simulink model "sampleModel7126_pp_1_1"  (R2018a)
settings: Solver=VariableStepAuto  StartTime=0.0  StopTime=10.0  RelTol=1e-3
undefined symbols (not defined in the file): DiscIntNeverNeededParam
libraries: simulink x367
(part 5 of 12)

== system sampleModel7126_pp_1_1/cfblk284 ==
  cfblk1 : Inport
  cfblk8 : Inport  Port=2
  Action Port : ActionPort  ActionType=else
  cfblk10 : Subsystem  TreatAsAtomicUnit=on
  cfblk11 : Subsystem  TreatAsAtomicUnit=on
  cfblk12 : Subsystem  TreatAsAtomicUnit=on
  cfblk{5,13..14,16} (4 alike) : Delay
  cfblk15 : Subsystem  TreatAsAtomicUnit=on
  cfblk3 : Subsystem  TreatAsAtomicUnit=on
  cfblk4 : simulink/Continuous/PID Controller (2DOF)  Controller=PID  TimeDomain=Discrete-time  SampleTime=-1  IntegratorMethod=Forward Euler  FilterMethod=Forward Euler  Form=Parallel  UseFilter=on  ControllerParametersSource=internal  P=1  I=1  D=0  N=100  b=1  c=1  InitialConditionSource=internal  InitialConditionForIntegrator=0  InitialConditionForFilter=0  ExternalReset=none  LimitOutput=off  UpperSaturationLimit=inf  LowerSaturationLimit=-inf  LinearizeAsGain=off  AntiWindupMode=none  Kb=1  TrackingMode=off  Kt=1  PParamMin=[]  PParamMax=[]  IParamMin=[]  IParamMax=[]  DParamMin=[]  DParamMax=[]  NParamMin=[]  NParamMax=[]  bParamMin=[]  bParamMax=[]  cParamMin=[]  cParamMax=[]  KbParamMin=[]  KbParamMax=[]  KtParamMin=[]  KtParamMax=[]  POutMin=[]  POutMax=[]  IOutMin=[]  IOutMax=[]  DOutMin=[]  DOutMax=[]  NOutMin=[]  NOutMax=[]  bOutMin=[]  bOutMax=[]  cOutMin=[]  cOutMax=[]  KbOutMin=[]  KbOutMax=[]  KtOutMin=[]  KtOutMax=[]  IntegratorOutMin=[]  IntegratorOutMax=[]  FilterOutMin=[]  FilterOutMax=[]  SumOutMin=[]  SumOutMax=[]  Sum1OutMin=[]  Sum1OutMax=[]  Sum2OutMin=[]  Sum2OutMax=[]  Sum3OutMin=[]  Sum3OutMax=[]  SumI1OutMin=[]  SumI1OutMax=[]  SumI2OutMin=[]  SumI2OutMax=[]  SumI3OutMin=[]  SumI3OutMax=[]  SumDOutMin=[]  SumDOutMax=[]  SaturationOutMin=[]  SaturationOutMax=[]  IntegratorContinuousStateAttributes=''  IntegratorStateMustResolveToSignalObject=off  IntegratorRTWStateStorageClass=Auto  FilterContinuousStateAttributes=''  FilterStateMustResolveToSignalObject=off  FilterRTWStateStorageClass=Auto  DifferentiatorICPrevScaledInput=0  DifferentiatorOutMin=[]  DifferentiatorOutMax=[]  FilterDiffOutCoefMin=[]  FilterDiffOutCoefMax=[]  SumDenOutMin=[]  SumDenOutMax=[]  SumNumOutMin=[]  SumNumOutMax=[]  ReciprocalOutMin=[]  ReciprocalOutMax=[]  DivideOutMin=[]  DivideOutMax=[]  TunerSelectOption=Transfer Function Based (PID Tuner App)
  cfblk6 : Delay  DelayLengthSource=Input port
      settings: InputPortMap=u0,p1
  cfblk7 : If  SampleTime=1
  cyemi_{1015..1018,1026..1028,1043..1054} (19 alike) : DataTypeConversion  OutDataTypeStr=double
  emi_1219 : Subsystem  TreatAsAtomicUnit=on
  emi_1221 : If  IfExpression=0 <= u1
  emi_1222 : DataTypeConversion  OutDataTypeStr=double
  emi_1655 : Subsystem  TreatAsAtomicUnit=on
  emi_1657 : If  IfExpression=0 <= u1  SampleTime=[1 0]
  emi_1658 : DataTypeConversion  OutDataTypeStr=double
  emi_2001 : Subsystem  TreatAsAtomicUnit=on
  emi_2003 : If  IfExpression=0 <= u1  SampleTime=[1 0]
  emi_2004 : DataTypeConversion  OutDataTypeStr=double
  cfblk2 : Outport
  cfblk9 : Outport  Port=2
  wires:
  cfblk8/1 -> cyemi_1016/1, cyemi_1048/1
  cfblk5/1 -> cfblk2/1, cyemi_1044/1, emi_1222/1
  cfblk4/1 -> cyemi_1043/1, cyemi_1046/1, cyemi_1047/1
  cfblk10/2(cfblk13) -> cfblk9/1
  cfblk7/1 -> cfblk10/Action
  cfblk7/2 -> cfblk11/Action
  cyemi_1015/1 -> cfblk10/1(cfblk1)
  cfblk14/1 -> cyemi_1015/1
  cyemi_1016/1 -> cfblk10/2(cfblk10)
  cyemi_1017/1 -> cfblk10/3(cfblk11)
  cfblk16/1 -> cyemi_1017/1
  cyemi_1018/1 -> cfblk10/4(cfblk12)
  cfblk13/1 -> cyemi_1018/1
  cyemi_1026/1 -> cfblk11/1(cfblk1)
  cyemi_1027/1 -> cfblk11/2(cfblk13)
  cfblk10/4(cfblk15) -> cyemi_1027/1
  cyemi_1028/1 -> cfblk11/3(cfblk14)
  cyemi_1044/1 -> cfblk13/1
  cyemi_1045/1 -> cfblk14/1
  cfblk11/2(cfblk15) -> cyemi_1045/1
  cyemi_1047/1 -> cfblk16/1
  cyemi_1049/1 -> cfblk4/1
  cfblk10/1(cfblk2) -> cyemi_1049/1
  cyemi_1050/1 -> cfblk4/2
  cfblk10/3(cfblk14) -> cyemi_1050/1
  cyemi_1051/1 -> cfblk5/1
  cfblk6/1 -> cyemi_1051/1, emi_1658/1, emi_2004/1
  cyemi_1052/1 -> cfblk6/1
  cyemi_1053/1 -> cfblk6/2
  cfblk11/1(cfblk2) -> cyemi_1053/1
  cyemi_1054/1 -> cfblk7/1
  cfblk1/1 -> cyemi_1054/1
  cyemi_1043/1 -> cfblk12/1(emi_1217)
  cfblk12/1(emi_1218) -> cyemi_1026/1
  emi_1221/1 -> cfblk12/Action
  emi_1221/2 -> emi_1219/Action
  emi_1222/1 -> emi_1221/1
  cyemi_1048/1 -> cfblk3/1(emi_1653)
  cfblk3/1(emi_1654) -> cyemi_1052/1
  emi_1657/1 -> cfblk3/Action
  emi_1657/2 -> emi_1655/Action
  emi_1658/1 -> emi_1657/1
  cyemi_1046/1 -> cfblk15/1(emi_1999)
  cfblk15/1(emi_2000) -> cyemi_1028/1
  emi_2003/1 -> cfblk15/Action
  emi_2003/2 -> emi_2001/Action
  emi_2004/1 -> emi_2003/1

== system sampleModel7126_pp_1_1/cfblk285 ==
  cfblk1 : Inport
  cfblk8 : Inport  Port=2
  cfblk9 : Inport  Port=3
  Action Port : ActionPort  ActionType=then
  cfblk3 : DiscreteZeroPole  Poles=[0 0.5]  Gain=1  SampleTime=-1
  cfblk4 : simulink/Discrete/Tapped Delay  vinit=0.0  samptime=-1  NumDelays=1  DelayOrder=Oldest  includeCurrent=off
  cfblk5 : simulink/Discrete/Transfer Fcn Lead or Lag  PoleZ=0.95  ZeroZ=0.75  ICPrevOutput=0.0  ICPrevInput=0.0  DoSatur=off
      settings: SourceProductName=Simulink  SourceProductBaseCode=SL
  cfblk6 : Subsystem  TreatAsAtomicUnit=on
  cfblk7 : DiscreteTransferFcn
  cyemi_{1058..1062} (5 alike) : DataTypeConversion  OutDataTypeStr=double
  emi_762 : Subsystem  TreatAsAtomicUnit=on
  emi_764 : If  IfExpression=Inf <= u1  SampleTime=[1 0]
  emi_765 : DataTypeConversion  OutDataTypeStr=double
  cfblk2 : Outport
  wires:
  cfblk3/1 -> cfblk2/1, emi_765/1
  cyemi_1058/1 -> cfblk3/1
  cyemi_1059/1 -> cfblk4/1
  cfblk7/1 -> cyemi_1059/1
  cyemi_1060/1 -> cfblk5/1
  cfblk1/1 -> cyemi_1060/1
  cfblk9/1 -> cyemi_1061/1
  cyemi_1062/1 -> cfblk7/1
  cfblk5/1 -> cyemi_1062/1
  cyemi_1061/1 -> cfblk6/1(emi_760)
  cfblk6/1(emi_761) -> cyemi_1058/1
  emi_764/1 -> cfblk6/Action
  emi_764/2 -> emi_762/Action
  emi_765/1 -> emi_764/1

== system sampleModel7126_pp_1_1/cfblk286 ==
  cfblk1 : Inport
  cfblk7 : Inport  Port=2
  cfblk8 : Inport  Port=3
  Action Port : ActionPort  ActionType=else
  cfblk3 : simulink/Discrete/Difference  ICPrevInput=0.0  OutMin=[]  OutMax=[]  OutDataTypeStr=double  OutputDataTypeScalingMode=double  OutDataType=fixdt(1, 16)  OutScaling=2^-10  DoSatur=off
  cfblk4 : UnitDelay  SampleTime=-1
  cfblk5 : Subsystem  TreatAsAtomicUnit=on
  cfblk6 : DiscreteStateSpace  SampleTime=-1
  cyemi_1066 : DataTypeConversion  OutDataTypeStr=double
  cyemi_1067 : DataTypeConversion  OutDataTypeStr=uint8
  cyemi_1068 : DataTypeConversion  OutDataTypeStr=double
  cyemi_1069 : DataTypeConversion  OutDataTypeStr=double
  emi_734 : Subsystem  TreatAsAtomicUnit=on
  emi_736 : If  IfExpression=0 <= u1  SampleTime=[1 0]
  emi_737 : DataTypeConversion  OutDataTypeStr=uint8
  cfblk2 : Outport
  wires:
  cfblk4/1 -> cfblk2/1, emi_737/1
  cyemi_1066/1 -> cfblk3/1
  cyemi_1067/1 -> cfblk4/1
  cfblk1/1 -> cyemi_1067/1
  cfblk8/1 -> cyemi_1068/1
  cyemi_1069/1 -> cfblk6/1
  cfblk7/1 -> cyemi_1069/1
  cyemi_1068/1 -> cfblk5/1(emi_732)
  cfblk5/1(emi_733) -> cyemi_1066/1
  emi_736/1 -> cfblk5/Action
  emi_736/2 -> emi_734/Action
  emi_737/1 -> emi_736/1

== system sampleModel7126_pp_1_1/cfblk287 ==
  cfblk1 : Inport
  cfblk8 : Inport  Port=2
  cfblk9 : Inport  Port=3
  Action Port : ActionPort  ActionType=then
  cfblk10 : Delay
  cfblk3 : simulink/Continuous/PID Controller (2DOF)  Controller=PID  TimeDomain=Discrete-time  SampleTime=-1  IntegratorMethod=Forward Euler  FilterMethod=Forward Euler  Form=Parallel  UseFilter=on  ControllerParametersSource=internal  P=1  I=1  D=0  N=100  b=1  c=1  InitialConditionSource=internal  InitialConditionForIntegrator=0  InitialConditionForFilter=0  ExternalReset=none  LimitOutput=off  UpperSaturationLimit=inf  LowerSaturationLimit=-inf  LinearizeAsGain=off  AntiWindupMode=none  Kb=1  TrackingMode=off  Kt=1  PParamMin=[]  PParamMax=[]  IParamMin=[]  IParamMax=[]  DParamMin=[]  DParamMax=[]  NParamMin=[]  NParamMax=[]  bParamMin=[]  bParamMax=[]  cParamMin=[]  cParamMax=[]  KbParamMin=[]  KbParamMax=[]  KtParamMin=[]  KtParamMax=[]  POutMin=[]  POutMax=[]  IOutMin=[]  IOutMax=[]  DOutMin=[]  DOutMax=[]  NOutMin=[]  NOutMax=[]  bOutMin=[]  bOutMax=[]  cOutMin=[]  cOutMax=[]  KbOutMin=[]  KbOutMax=[]  KtOutMin=[]  KtOutMax=[]  IntegratorOutMin=[]  IntegratorOutMax=[]  FilterOutMin=[]  FilterOutMax=[]  SumOutMin=[]  SumOutMax=[]  Sum1OutMin=[]  Sum1OutMax=[]  Sum2OutMin=[]  Sum2OutMax=[]  Sum3OutMin=[]  Sum3OutMax=[]  SumI1OutMin=[]  SumI1OutMax=[]  SumI2OutMin=[]  SumI2OutMax=[]  SumI3OutMin=[]  SumI3OutMax=[]  SumDOutMin=[]  SumDOutMax=[]  SaturationOutMin=[]  SaturationOutMax=[]  IntegratorContinuousStateAttributes=''  IntegratorStateMustResolveToSignalObject=off  IntegratorRTWStateStorageClass=Auto  FilterContinuousStateAttributes=''  FilterStateMustResolveToSignalObject=off  FilterRTWStateStorageClass=Auto  DifferentiatorICPrevScaledInput=0  DifferentiatorOutMin=[]  DifferentiatorOutMax=[]  FilterDiffOutCoefMin=[]  FilterDiffOutCoefMax=[]  SumDenOutMin=[]  SumDenOutMax=[]  SumNumOutMin=[]  SumNumOutMax=[]  ReciprocalOutMin=[]  ReciprocalOutMax=[]  DivideOutMin=[]  DivideOutMax=[]  TunerSelectOption=Transfer Function Based (PID Tuner App)
  cfblk4 : Subsystem  TreatAsAtomicUnit=on
  cfblk5 : DiscreteIntegrator  SampleTime=-1  OutDataTypeStr=double  ICPrevOutput=DiscIntNeverNeededParam  ICPrevScaledInput=DiscIntNeverNeededParam
  cfblk6 : Subsystem  TreatAsAtomicUnit=on
  cfblk7 : Subsystem  TreatAsAtomicUnit=on
  cyemi_{1073..1080} (8 alike) : DataTypeConversion  OutDataTypeStr=double
  emi_1677 : Subsystem  TreatAsAtomicUnit=on
  emi_1679 : If  IfExpression=Inf <= u1  SampleTime=[1 0]
  emi_1680 : DataTypeConversion  OutDataTypeStr=double
  emi_720 : Subsystem  TreatAsAtomicUnit=on
  emi_722 : If  IfExpression=Inf <= u1  SampleTime=[1 0]
  emi_723 : DataTypeConversion  OutDataTypeStr=double
  emi_755 : Subsystem  TreatAsAtomicUnit=on
  emi_757 : If  IfExpression=Inf <= u1  SampleTime=[1 0]
  emi_758 : DataTypeConversion  OutDataTypeStr=double
  cfblk2 : Outport
  wires:
  cfblk5/1 -> cfblk2/1, emi_1680/1
  cyemi_1073/1 -> cfblk10/1
  cyemi_1074/1 -> cfblk3/1
  cfblk10/1 -> cyemi_1074/1
  cyemi_1075/1 -> cfblk3/2
  cfblk9/1 -> cyemi_1075/1
  cfblk3/1 -> cyemi_1076/1
  cyemi_1077/1 -> cfblk5/1
  cfblk1/1 -> cyemi_1078/1
  cfblk8/1 -> cyemi_1080/1
  cyemi_1076/1 -> cfblk4/1(emi_718)
  cfblk4/1(emi_719) -> cyemi_1073/1
  emi_722/1 -> cfblk4/Action
  emi_722/2 -> emi_720/Action
  emi_723/1 -> emi_722/1
  cyemi_1078/1 -> cfblk6/1(emi_753)
  cfblk6/1(emi_754) -> cyemi_1079/1
  emi_757/1 -> cfblk6/Action
  emi_757/2 -> emi_755/Action
  emi_758/1 -> emi_757/1
  cyemi_1079/1 -> cfblk7/1(emi_1674)
  cyemi_1080/1 -> cfblk7/2(emi_1675)
  cfblk7/1(emi_1676) -> emi_758/1, emi_723/1, cyemi_1077/1
  emi_1679/1 -> cfblk7/Action
  emi_1679/2 -> emi_1677/Action
  emi_1680/1 -> emi_1679/1

== system sampleModel7126_pp_1_1/cfblk288 ==
  cfblk1 : Inport
  cfblk13 : Inport  Port=2
  Action Port : ActionPort  ActionType=else
  cfblk10 : simulink/Discrete/Tapped Delay  vinit=0.0  samptime=-1  NumDelays=1  DelayOrder=Oldest  includeCurrent=off
  cfblk11 : Subsystem  TreatAsAtomicUnit=on
  cfblk12 : DiscreteStateSpace  SampleTime=-1
  cfblk3 : Subsystem  TreatAsAtomicUnit=on
  cfblk4 : UnitDelay  SampleTime=-1
  cfblk5 : DiscreteFir
  cfblk6 : Delay  ShowEnablePort=on
      settings: InputPortMap=u0,e6
  cfblk7 : simulink/Discrete/Transfer Fcn First Order  PoleZ=0.95  ICPrevOutput=0.0  DoSatur=off
      settings: SourceProductName=Simulink
  cfblk8 : simulink/Continuous/PID Controller  Controller=PID  TimeDomain=Discrete-time  SampleTime=-1  IntegratorMethod=Forward Euler  FilterMethod=Forward Euler  Form=Parallel  UseFilter=on  ControllerParametersSource=internal  P=1  I=1  D=0  N=100  InitialConditionSource=internal  InitialConditionForIntegrator=0  InitialConditionForFilter=0  ExternalReset=none  LimitOutput=off  UpperSaturationLimit=inf  LowerSaturationLimit=-inf  LinearizeAsGain=off  AntiWindupMode=none  Kb=1  TrackingMode=off  Kt=1  PParamMin=[]  PParamMax=[]  IParamMin=[]  IParamMax=[]  DParamMin=[]  DParamMax=[]  NParamMin=[]  NParamMax=[]  KbParamMin=[]  KbParamMax=[]  KtParamMin=[]  KtParamMax=[]  POutMin=[]  POutMax=[]  IOutMin=[]  IOutMax=[]  DOutMin=[]  DOutMax=[]  NOutMin=[]  NOutMax=[]  KbOutMin=[]  KbOutMax=[]  KtOutMin=[]  KtOutMax=[]  IntegratorOutMin=[]  IntegratorOutMax=[]  FilterOutMin=[]  FilterOutMax=[]  SumOutMin=[]  SumOutMax=[]  SumI1OutMin=[]  SumI1OutMax=[]  SumI2OutMin=[]  SumI2OutMax=[]  SumI3OutMin=[]  SumI3OutMax=[]  SumDOutMin=[]  SumDOutMax=[]  SaturationOutMin=[]  SaturationOutMax=[]  IntegratorContinuousStateAttributes=''  IntegratorStateMustResolveToSignalObject=off  IntegratorRTWStateStorageClass=Auto  FilterContinuousStateAttributes=''  FilterStateMustResolveToSignalObject=off  FilterRTWStateStorageClass=Auto  DifferentiatorICPrevScaledInput=0  DifferentiatorOutMin=[]  DifferentiatorOutMax=[]  FilterDiffOutCoefMin=[]  FilterDiffOutCoefMax=[]  SumDenOutMin=[]  SumDenOutMax=[]  SumNumOutMin=[]  SumNumOutMax=[]  ReciprocalOutMin=[]  ReciprocalOutMax=[]  DivideOutMin=[]  DivideOutMax=[]  TunerSelectOption=Transfer Function Based (PID Tuner App)
  cfblk9 : DiscreteTransferFcn
  cyemi_{1083..1093} (11 alike) : DataTypeConversion  OutDataTypeStr=double
  emi_1350 : Subsystem  TreatAsAtomicUnit=on
  emi_1352 : If  IfExpression=0 <= u1  SampleTime=[1 0]
  emi_1353 : DataTypeConversion  OutDataTypeStr=double
  emi_346 : Subsystem  TreatAsAtomicUnit=on
  emi_348 : If  IfExpression=0 <= u1  SampleTime=[1 0]
  emi_349 : DataTypeConversion  OutDataTypeStr=double
  cfblk2 : Outport
  wires:
  cfblk12/1 -> cfblk2/1
  cyemi_1083/1 -> cfblk10/1
  cfblk8/1 -> cyemi_1083/1
  cfblk4/1 -> cyemi_1084/1
  cyemi_1085/1 -> cfblk12/1
  cfblk6/1 -> cyemi_1086/1, emi_349/1
  cyemi_1087/1 -> cfblk4/1
  cfblk7/1 -> cyemi_1087/1
  cyemi_1088/1 -> cfblk5/1
  cyemi_1089/1 -> cfblk6/1
  cfblk1/1 -> cyemi_1089/1
  cyemi_1090/1 -> cfblk6/2
  cfblk13/1 -> cyemi_1090/1
  cyemi_1091/1 -> cfblk7/1
  cfblk9/1 -> cyemi_1091/1
  cyemi_1092/1 -> cfblk8/1
  cfblk5/1 -> cyemi_1092/1
  cyemi_1093/1 -> cfblk9/1
  cfblk10/1 -> cyemi_1093/1, emi_1353/1
  cyemi_1084/1 -> cfblk11/1(emi_344)
  cfblk11/1(emi_345) -> cyemi_1085/1
  emi_348/1 -> cfblk11/Action
  emi_348/2 -> emi_346/Action
  emi_349/1 -> emi_348/1
  cyemi_1086/1 -> cfblk3/1(emi_1348)
  cfblk3/1(emi_1349) -> cyemi_1088/1
  emi_1352/1 -> cfblk3/Action
  emi_1352/2 -> emi_1350/Action
  emi_1353/1 -> emi_1352/1

== system sampleModel7126_pp_1_1/cfblk289 ==
  cfblk1 : Inport
  Action Port : ActionPort  ActionType=then
  cfblk10 : Subsystem  TreatAsAtomicUnit=on
  cfblk11 : Subsystem  TreatAsAtomicUnit=on
  cfblk12 : Delay
  cfblk3 : simulink/Discrete/Transfer Fcn First Order  PoleZ=0.95  ICPrevOutput=0.0  DoSatur=off
      settings: SourceProductName=Simulink
  cfblk4 : DiscreteStateSpace  SampleTime=-1
  cfblk5 : simulink/Discrete/Transfer Fcn Real Zero  ZeroZ=0.75  ICPrevInput=0.0  DoSatur=off
      settings: SourceProductName=Simulink  SourceProductBaseCode=SL
  cfblk6 : DiscreteZeroPole  Poles=[0 0.5]  Gain=1  SampleTime=-1
  cfblk7 : If  SampleTime=1
  cfblk9 : Subsystem  TreatAsAtomicUnit=on
  cyemi_{1095..1096,1108..1116} (11 alike) : DataTypeConversion  OutDataTypeStr=double
  emi_1126 : Subsystem  TreatAsAtomicUnit=on
  emi_1128 : If  IfExpression=Inf <= u1
  emi_1129 : DataTypeConversion  OutDataTypeStr=double
  cfblk2 : Outport
  cfblk8 : Outport  Port=2
  wires:
  cfblk4/1 -> cyemi_1114/1, cyemi_1115/1, cyemi_1116/1, emi_1129/1
  cfblk6/1 -> cfblk2/1
  cfblk1/1 -> cfblk8/1, cyemi_1110/1
  cfblk7/1 -> cfblk9/Action
  cfblk7/2 -> cfblk10/Action
  cyemi_1095/1 -> cfblk10/1(cfblk1)
  cfblk3/1 -> cyemi_1095/1
  cyemi_1096/1 -> cfblk10/2(cfblk12)
  cfblk5/1 -> cyemi_1108/1
  cyemi_1109/1 -> cfblk12/1
  cfblk9/2(cfblk17) -> cyemi_1109/1
  cyemi_1110/1 -> cfblk3/1
  cyemi_1111/1 -> cfblk4/1
  cfblk12/1 -> cyemi_1111/1
  cyemi_1112/1 -> cfblk5/1
  cfblk10/1(cfblk2) -> cyemi_1112/1
  cyemi_1113/1 -> cfblk6/1
  cfblk9/1(cfblk2) -> cyemi_1113/1
  cyemi_1114/1 -> cfblk7/1
  cyemi_1115/1 -> cfblk9/1(cfblk1)
  cyemi_1116/1 -> cfblk9/2(cfblk16)
  cyemi_1108/1 -> cfblk11/1(emi_1124)
  cfblk11/1(emi_1125) -> cyemi_1096/1
  emi_1128/1 -> cfblk11/Action
  emi_1128/2 -> emi_1126/Action
  emi_1129/1 -> emi_1128/1

== system sampleModel7126_pp_1_1/cfblk290 ==
  cfblk1 : Inport
  cfblk10 : Inport  Port=2
  cfblk11 : Inport  Port=3
  cfblk12 : Inport  Port=4
  Action Port : ActionPort  ActionType=else
  cfblk3 : Subsystem  TreatAsAtomicUnit=on
  cfblk4 : simulink/Discrete/Transfer Fcn Real Zero  ZeroZ=0.75  ICPrevInput=0.0  DoSatur=off
      settings: SourceProductName=Simulink  SourceProductBaseCode=SL
  cfblk5 : Subsystem  TreatAsAtomicUnit=on
  cfblk6 : Subsystem  TreatAsAtomicUnit=on
  cfblk7 : Subsystem  TreatAsAtomicUnit=on
  cfblk8 : Subsystem  TreatAsAtomicUnit=on
  cfblk9 : DiscreteStateSpace  SampleTime=-1
  cyemi_{1138..1140,1142..1145} (7 alike) : DataTypeConversion  OutDataTypeStr=double
  cyemi_1141 : DataTypeConversion  OutDataTypeStr=uint8
  emi_1154 : Subsystem  TreatAsAtomicUnit=on
  emi_{1156,1243,1387,1874} (4 alike) : If  IfExpression=0 <= u1  SampleTime=[1 0]
  emi_{1157,1244,1388,1730,1875} (5 alike) : DataTypeConversion  OutDataTypeStr=double
  emi_1241 : Subsystem  TreatAsAtomicUnit=on
  emi_1385 : Subsystem  TreatAsAtomicUnit=on
  emi_1727 : Subsystem  TreatAsAtomicUnit=on
  emi_1729 : If  IfExpression=0 <= u1
  emi_1872 : Subsystem  TreatAsAtomicUnit=on
  cfblk2 : Outport
  cfblk13 : Outport  Port=2
  cfblk14 : Outport  Port=3
  cfblk15 : Outport  Port=4
  cfblk16 : Outport  Port=5
  wires:
  cfblk1/1 -> cfblk15/1
  cfblk4/1 -> cyemi_1138/1, cyemi_1142/1
  cyemi_1139/1 -> cfblk4/1
  cfblk9/1 -> cyemi_1140/1, emi_1157/1
  cfblk10/1 -> cyemi_1141/1
  cfblk11/1 -> cyemi_1143/1
  cfblk12/1 -> cyemi_1144/1
  cyemi_1145/1 -> cfblk9/1
  cyemi_1144/1 -> cfblk8/1(emi_1152)
  cfblk8/1(emi_1153) -> cyemi_1145/1, emi_1875/1
  emi_1156/1 -> cfblk8/Action
  emi_1156/2 -> emi_1154/Action
  emi_1157/1 -> emi_1156/1
  cyemi_1140/1 -> cfblk5/1(emi_1239)
  cfblk5/1(emi_1240) -> cyemi_1139/1, emi_1730/1
  emi_1243/1 -> cfblk5/Action
  emi_1243/2 -> emi_1241/Action
  emi_1244/1 -> emi_1243/1
  cyemi_1143/1 -> cfblk7/1(emi_1383)
  cfblk7/1(emi_1384) -> cfblk14/1
  emi_1387/1 -> cfblk7/Action
  emi_1387/2 -> emi_1385/Action
  emi_1388/1 -> emi_1387/1
  cyemi_1138/1 -> cfblk3/1(emi_1725)
  cfblk3/1(emi_1726) -> emi_1388/1, emi_1244/1, cfblk13/1
  emi_1729/1 -> cfblk3/Action
  emi_1729/2 -> emi_1727/Action
  emi_1730/1 -> emi_1729/1
  cyemi_1141/1 -> cfblk6/1(emi_1869)
  cyemi_1142/1 -> cfblk6/2(emi_1870)
  cfblk6/1(emi_1871) -> cfblk16/1, cfblk2/1
  emi_1874/1 -> cfblk6/Action
  emi_1874/2 -> emi_1872/Action
  emi_1875/1 -> emi_1874/1

== system sampleModel7126_pp_1_1/cfblk291 ==
  cfblk1 : Inport
  Action Port : ActionPort  ActionType=then
  cfblk3 : DiscreteTransferFcn
  cfblk4 : Delay  ShowEnablePort=on
      settings: InputPortMap=u0,e6
  cfblk5 : DiscreteZeroPole  Poles=[0 0.5]  Gain=1  SampleTime=-1
  cfblk6 : Subsystem  TreatAsAtomicUnit=on
  cfblk7 : DiscreteFilter
  cyemi_{1147..1153} (7 alike) : DataTypeConversion  OutDataTypeStr=double
  emi_432 : Subsystem  TreatAsAtomicUnit=on
  emi_434 : If  IfExpression=Inf <= u1  SampleTime=[1 0]
  emi_435 : DataTypeConversion  OutDataTypeStr=double
  cfblk2 : Outport
  cfblk8 : Outport  Port=2
  wires:
  cfblk1/1 -> cfblk8/1, cyemi_1147/1, cyemi_1149/1, cyemi_1150/1
  cyemi_1147/1 -> cfblk3/1
  cyemi_1148/1 -> cfblk4/1
  cfblk3/1 -> cyemi_1148/1
  cyemi_1149/1 -> cfblk4/2
  cyemi_1150/1 -> cfblk5/1
  cfblk7/1 -> cyemi_1151/1
  cfblk4/1 -> cyemi_1152/1
  cyemi_1153/1 -> cfblk7/1
  cfblk5/1 -> cyemi_1153/1, emi_435/1
  cyemi_1151/1 -> cfblk6/1(emi_429)
  cyemi_1152/1 -> cfblk6/2(emi_430)
  cfblk6/1(emi_431) -> cfblk2/1
  emi_434/1 -> cfblk6/Action
  emi_434/2 -> emi_432/Action
  emi_435/1 -> emi_434/1

== system sampleModel7126_pp_1_1/cfblk292 ==
  cfblk1 : Inport
  cfblk11 : Inport  Port=2
  Action Port : ActionPort  ActionType=else
  cfblk10 : If  SampleTime=1
  cfblk14 : Subsystem  TreatAsAtomicUnit=on
  cfblk15 : Subsystem  TreatAsAtomicUnit=on
  cfblk16 : Subsystem  TreatAsAtomicUnit=on
  cfblk17 : Delay
  cfblk3 : UnitDelay  SampleTime=-1
  cfblk4 : Delay  ShowEnablePort=on
      settings: InputPortMap=u0,e6
  cfblk5 : simulink/Discrete/Transfer Fcn Lead or Lag  PoleZ=0.95  ZeroZ=0.75  ICPrevOutput=0.0  ICPrevInput=0.0  DoSatur=off
      settings: SourceProductName=Simulink  SourceProductBaseCode=SL
  cfblk6 : Subsystem  TreatAsAtomicUnit=on
  cfblk7 : simulink/Continuous/PID Controller  Controller=PID  TimeDomain=Discrete-time  SampleTime=-1  IntegratorMethod=Forward Euler  FilterMethod=Forward Euler  Form=Parallel  UseFilter=on  ControllerParametersSource=internal  P=1  I=1  D=0  N=100  InitialConditionSource=internal  InitialConditionForIntegrator=0  InitialConditionForFilter=0  ExternalReset=none  LimitOutput=off  UpperSaturationLimit=inf  LowerSaturationLimit=-inf  LinearizeAsGain=off  AntiWindupMode=none  Kb=1  TrackingMode=off  Kt=1  PParamMin=[]  PParamMax=[]  IParamMin=[]  IParamMax=[]  DParamMin=[]  DParamMax=[]  NParamMin=[]  NParamMax=[]  KbParamMin=[]  KbParamMax=[]  KtParamMin=[]  KtParamMax=[]  POutMin=[]  POutMax=[]  IOutMin=[]  IOutMax=[]  DOutMin=[]  DOutMax=[]  NOutMin=[]  NOutMax=[]  KbOutMin=[]  KbOutMax=[]  KtOutMin=[]  KtOutMax=[]  IntegratorOutMin=[]  IntegratorOutMax=[]  FilterOutMin=[]  FilterOutMax=[]  SumOutMin=[]  SumOutMax=[]  SumI1OutMin=[]  SumI1OutMax=[]  SumI2OutMin=[]  SumI2OutMax=[]  SumI3OutMin=[]  SumI3OutMax=[]  SumDOutMin=[]  SumDOutMax=[]  SaturationOutMin=[]  SaturationOutMax=[]  IntegratorContinuousStateAttributes=''  IntegratorStateMustResolveToSignalObject=off  IntegratorRTWStateStorageClass=Auto  FilterContinuousStateAttributes=''  FilterStateMustResolveToSignalObject=off  FilterRTWStateStorageClass=Auto  DifferentiatorICPrevScaledInput=0  DifferentiatorOutMin=[]  DifferentiatorOutMax=[]  FilterDiffOutCoefMin=[]  FilterDiffOutCoefMax=[]  SumDenOutMin=[]  SumDenOutMax=[]  SumNumOutMin=[]  SumNumOutMax=[]  ReciprocalOutMin=[]  ReciprocalOutMax=[]  DivideOutMin=[]  DivideOutMax=[]  TunerSelectOption=Transfer Function Based (PID Tuner App)
  cfblk8 : simulink/Continuous/PID Controller  Controller=PID  TimeDomain=Discrete-time  SampleTime=-1  IntegratorMethod=Forward Euler  FilterMethod=Forward Euler  Form=Parallel  UseFilter=on  ControllerParametersSource=internal  P=1  I=1  D=0  N=100  InitialConditionSource=internal  InitialConditionForIntegrator=0  InitialConditionForFilter=0  ExternalReset=none  LimitOutput=off  UpperSaturationLimit=inf  LowerSaturationLimit=-inf  LinearizeAsGain=off  AntiWindupMode=none  Kb=1  TrackingMode=off  Kt=1  PParamMin=[]  PParamMax=[]  IParamMin=[]  IParamMax=[]  DParamMin=[]  DParamMax=[]  NParamMin=[]  NParamMax=[]  KbParamMin=[]  KbParamMax=[]  KtParamMin=[]  KtParamMax=[]  POutMin=[]  POutMax=[]  IOutMin=[]  IOutMax=[]  DOutMin=[]  DOutMax=[]  NOutMin=[]  NOutMax=[]  KbOutMin=[]  KbOutMax=[]  KtOutMin=[]  KtOutMax=[]  IntegratorOutMin=[]  IntegratorOutMax=[]  FilterOutMin=[]  FilterOutMax=[]  SumOutMin=[]  SumOutMax=[]  SumI1OutMin=[]  SumI1OutMax=[]  SumI2OutMin=[]  SumI2OutMax=[]  SumI3OutMin=[]  SumI3OutMax=[]  SumDOutMin=[]  SumDOutMax=[]  SaturationOutMin=[]  SaturationOutMax=[]  IntegratorContinuousStateAttributes=''  IntegratorStateMustResolveToSignalObject=off  IntegratorRTWStateStorageClass=Auto  FilterContinuousStateAttributes=''  FilterStateMustResolveToSignalObject=off  FilterRTWStateStorageClass=Auto  DifferentiatorICPrevScaledInput=0  DifferentiatorOutMin=[]  DifferentiatorOutMax=[]  FilterDiffOutCoefMin=[]  FilterDiffOutCoefMax=[]  SumDenOutMin=[]  SumDenOutMax=[]  SumNumOutMin=[]  SumNumOutMax=[]  ReciprocalOutMin=[]  ReciprocalOutMax=[]  DivideOutMin=[]  DivideOutMax=[]  TunerSelectOption=Transfer Function Based (PID Tuner App)
  cfblk9 : DiscreteTransferFcn
  cyemi_{1156..1157,1165..1168,1176..1185} (16 alike) : DataTypeConversion  OutDataTypeStr=double
  emi_1112 : Subsystem  TreatAsAtomicUnit=on
  emi_1114 : If  IfExpression=0 <= u1  SampleTime=[1 0]
  emi_1115 : DataTypeConversion  OutDataTypeStr=double
  emi_303 : Subsystem  TreatAsAtomicUnit=on
  emi_305 : If  IfExpression=0 <= u1  SampleTime=[1 0]
  emi_306 : DataTypeConversion  OutDataTypeStr=double
  cfblk2 : Outport
  cfblk12 : Outport  Port=2
  cfblk13 : Outport  Port=3
  wires:
  cfblk8/1 -> cyemi_1176/1, cyemi_1178/1
  cfblk1/1 -> cyemi_1156/1, cyemi_1183/1
  cfblk3/1 -> cfblk12/1, emi_306/1
  cfblk7/1 -> cfblk13/1
  cfblk15/1(cfblk2) -> cfblk2/1
  cfblk14/2(cfblk7) -> cyemi_1168/1, cyemi_1181/1
  cfblk10/1 -> cfblk14/Action
  cfblk10/2 -> cfblk15/Action
  cyemi_1156/1 -> cfblk10/1
  cyemi_1157/1 -> cfblk14/1(cfblk1)
  cfblk17/1 -> cyemi_1157/1
  cyemi_1165/1 -> cfblk15/1(cfblk1)
  cfblk14/1(cfblk2) -> cyemi_1165/1
  cyemi_1166/1 -> cfblk15/2(cfblk8)
  cfblk11/1 -> cyemi_1166/1
  cyemi_1167/1 -> cfblk15/3(cfblk9)
  cyemi_1168/1 -> cfblk15/4(cfblk10)
  cyemi_1177/1 -> cfblk17/1
  cfblk15/3(cfblk12) -> cyemi_1177/1
  cyemi_1178/1 -> cfblk3/1
  cyemi_1179/1 -> cfblk4/1
  cfblk5/1 -> cyemi_1179/1
  cyemi_1180/1 -> cfblk4/2
  cfblk9/1 -> cyemi_1180/1, emi_1115/1
  cyemi_1181/1 -> cfblk5/1
  cfblk4/1 -> cyemi_1182/1
  cyemi_1183/1 -> cfblk7/1
  cyemi_1184/1 -> cfblk8/1
  cyemi_1185/1 -> cfblk9/1
  cfblk15/2(cfblk11) -> cyemi_1185/1
  cyemi_1176/1 -> cfblk16/1(emi_301)
  cfblk16/1(emi_302) -> cyemi_1167/1
  emi_305/1 -> cfblk16/Action
  emi_305/2 -> emi_303/Action
  emi_306/1 -> emi_305/1
  cyemi_1182/1 -> cfblk6/1(emi_1110)
  cfblk6/1(emi_1111) -> cyemi_1184/1
  emi_1114/1 -> cfblk6/Action
  emi_1114/2 -> emi_1112/Action
  emi_1115/1 -> emi_1114/1

== system sampleModel7126_pp_1_1/cfblk293 ==
  cfblk1 : Inport
  cfblk9 : Inport  Port=2
  Action Port : ActionPort  ActionType=then
  cfblk10 : Subsystem  TreatAsAtomicUnit=on
  cfblk11 : Delay
  cfblk12 : Subsystem  TreatAsAtomicUnit=on
  cfblk13 : Delay
  cfblk3 : simulink/Continuous/PID Controller (2DOF)  Controller=PID  TimeDomain=Discrete-time  SampleTime=-1  IntegratorMethod=Forward Euler  FilterMethod=Forward Euler  Form=Parallel  UseFilter=on  ControllerParametersSource=internal  P=1  I=1  D=0  N=100  b=1  c=1  InitialConditionSource=internal  InitialConditionForIntegrator=0  InitialConditionForFilter=0  ExternalReset=none  LimitOutput=off  UpperSaturationLimit=inf  LowerSaturationLimit=-inf  LinearizeAsGain=off  AntiWindupMode=none  Kb=1  TrackingMode=off  Kt=1  PParamMin=[]  PParamMax=[]  IParamMin=[]  IParamMax=[]  DParamMin=[]  DParamMax=[]  NParamMin=[]  NParamMax=[]  bParamMin=[]  bParamMax=[]  cParamMin=[]  cParamMax=[]  KbParamMin=[]  KbParamMax=[]  KtParamMin=[]  KtParamMax=[]  POutMin=[]  POutMax=[]  IOutMin=[]  IOutMax=[]  DOutMin=[]  DOutMax=[]  NOutMin=[]  NOutMax=[]  bOutMin=[]  bOutMax=[]  cOutMin=[]  cOutMax=[]  KbOutMin=[]  KbOutMax=[]  KtOutMin=[]  KtOutMax=[]  IntegratorOutMin=[]  IntegratorOutMax=[]  FilterOutMin=[]  FilterOutMax=[]  SumOutMin=[]  SumOutMax=[]  Sum1OutMin=[]  Sum1OutMax=[]  Sum2OutMin=[]  Sum2OutMax=[]  Sum3OutMin=[]  Sum3OutMax=[]  SumI1OutMin=[]  SumI1OutMax=[]  SumI2OutMin=[]  SumI2OutMax=[]  SumI3OutMin=[]  SumI3OutMax=[]  SumDOutMin=[]  SumDOutMax=[]  SaturationOutMin=[]  SaturationOutMax=[]  IntegratorContinuousStateAttributes=''  IntegratorStateMustResolveToSignalObject=off  IntegratorRTWStateStorageClass=Auto  FilterContinuousStateAttributes=''  FilterStateMustResolveToSignalObject=off  FilterRTWStateStorageClass=Auto  DifferentiatorICPrevScaledInput=0  DifferentiatorOutMin=[]  DifferentiatorOutMax=[]  FilterDiffOutCoefMin=[]  FilterDiffOutCoefMax=[]  SumDenOutMin=[]  SumDenOutMax=[]  SumNumOutMin=[]  SumNumOutMax=[]  ReciprocalOutMin=[]  ReciprocalOutMax=[]  DivideOutMin=[]  DivideOutMax=[]  TunerSelectOption=Transfer Function Based (PID Tuner App)
  cfblk4 : Subsystem  TreatAsAtomicUnit=on
  cfblk5 : Delay  ShowEnablePort=on
      settings: InputPortMap=u0,e6
  cfblk6 : Delay
  cfblk7 : simulink/Continuous/PID Controller (2DOF)  Controller=PID  TimeDomain=Discrete-time  SampleTime=-1  IntegratorMethod=Forward Euler  FilterMethod=Forward Euler  Form=Parallel  UseFilter=on  ControllerParametersSource=internal  P=1  I=1  D=0  N=100  b=1  c=1  InitialConditionSource=internal  InitialConditionForIntegrator=0  InitialConditionForFilter=0  ExternalReset=none  LimitOutput=off  UpperSaturationLimit=inf  LowerSaturationLimit=-inf  LinearizeAsGain=off  AntiWindupMode=none  Kb=1  TrackingMode=off  Kt=1  PParamMin=[]  PParamMax=[]  IParamMin=[]  IParamMax=[]  DParamMin=[]  DParamMax=[]  NParamMin=[]  NParamMax=[]  bParamMin=[]  bParamMax=[]  cParamMin=[]  cParamMax=[]  KbParamMin=[]  KbParamMax=[]  KtParamMin=[]  KtParamMax=[]  POutMin=[]  POutMax=[]  IOutMin=[]  IOutMax=[]  DOutMin=[]  DOutMax=[]  NOutMin=[]  NOutMax=[]  bOutMin=[]  bOutMax=[]  cOutMin=[]  cOutMax=[]  KbOutMin=[]  KbOutMax=[]  KtOutMin=[]  KtOutMax=[]  IntegratorOutMin=[]  IntegratorOutMax=[]  FilterOutMin=[]  FilterOutMax=[]  SumOutMin=[]  SumOutMax=[]  Sum1OutMin=[]  Sum1OutMax=[]  Sum2OutMin=[]  Sum2OutMax=[]  Sum3OutMin=[]  Sum3OutMax=[]  SumI1OutMin=[]  SumI1OutMax=[]  SumI2OutMin=[]  SumI2OutMax=[]  SumI3OutMin=[]  SumI3OutMax=[]  SumDOutMin=[]  SumDOutMax=[]  SaturationOutMin=[]  SaturationOutMax=[]  IntegratorContinuousStateAttributes=''  IntegratorStateMustResolveToSignalObject=off  IntegratorRTWStateStorageClass=Auto  FilterContinuousStateAttributes=''  FilterStateMustResolveToSignalObject=off  FilterRTWStateStorageClass=Auto  DifferentiatorICPrevScaledInput=0  DifferentiatorOutMin=[]  DifferentiatorOutMax=[]  FilterDiffOutCoefMin=[]  FilterDiffOutCoefMax=[]  SumDenOutMin=[]  SumDenOutMax=[]  SumNumOutMin=[]  SumNumOutMax=[]  ReciprocalOutMin=[]  ReciprocalOutMax=[]  DivideOutMin=[]  DivideOutMax=[]  TunerSelectOption=Transfer Function Based (PID Tuner App)
  cfblk8 : Subsystem  TreatAsAtomicUnit=on
  cyemi_{1188..1201} (14 alike) : DataTypeConversion  OutDataTypeStr=double
  emi_119 : Subsystem  TreatAsAtomicUnit=on
  emi_121 : If  IfExpression=Inf <= u1  SampleTime=[1 0]
  emi_{122,299,328,2178} (4 alike) : DataTypeConversion  OutDataTypeStr=double
  emi_2175 : Subsystem  TreatAsAtomicUnit=on
  emi_2177 : If  IfExpression=Inf <= u1
  emi_296 : Subsystem  TreatAsAtomicUnit=on
  emi_298 : If  IfExpression=Inf <= u1  SampleTime=[1 0]
  emi_325 : Subsystem  TreatAsAtomicUnit=on
  emi_327 : If  IfExpression=Inf <= u1  SampleTime=[1 0]
  cfblk2 : Outport
  wires:
  cfblk7/1 -> cyemi_1189/1, cyemi_1190/1, cyemi_1191/1
  cfblk1/1 -> cfblk2/1
  cyemi_1189/1 -> cfblk11/1
  cyemi_1191/1 -> cfblk13/1
  cyemi_1192/1 -> cfblk3/1
  cyemi_1193/1 -> cfblk3/2
  cfblk13/1 -> cyemi_1193/1, emi_299/1, emi_2178/1
  cfblk5/1 -> cyemi_1194/1
  cyemi_1196/1 -> cfblk5/1
  cfblk11/1 -> cyemi_1196/1
  cyemi_1197/1 -> cfblk5/2
  cfblk3/1 -> cyemi_1197/1
  cyemi_1198/1 -> cfblk6/1
  cyemi_1199/1 -> cfblk7/1
  cfblk9/1 -> cyemi_1199/1
  cyemi_1200/1 -> cfblk7/2
  cfblk6/1 -> cyemi_1201/1
  cyemi_1190/1 -> cfblk12/1(emi_117)
  cfblk12/1(emi_118) -> cyemi_1195/1
  emi_121/1 -> cfblk12/Action
  emi_121/2 -> emi_119/Action
  emi_122/1 -> emi_121/1
  cyemi_1201/1 -> cfblk8/1(emi_294)
  cfblk8/1(emi_295) -> cyemi_1200/1, cyemi_1188/1
  emi_298/1 -> cfblk8/Action
  emi_298/2 -> emi_296/Action
  emi_299/1 -> emi_298/1
  cyemi_1194/1 -> cfblk4/1(emi_322)
  cyemi_1195/1 -> cfblk4/2(emi_323)
  cfblk4/1(emi_324) -> cyemi_1198/1
  emi_327/1 -> cfblk4/Action
  emi_327/2 -> emi_325/Action
  emi_328/1 -> emi_327/1
  cyemi_1188/1 -> cfblk10/1(emi_2173)
  cfblk10/1(emi_2174) -> emi_328/1, emi_122/1, cyemi_1192/1
  emi_2177/1 -> cfblk10/Action
  emi_2177/2 -> emi_2175/Action
  emi_2178/1 -> emi_2177/1

== system sampleModel7126_pp_1_1/cfblk294 ==
  cfblk1 : Inport
  cfblk9 : Inport  Port=2
  cfblk10 : Inport  Port=3
  Action Port : ActionPort  ActionType=else
  cfblk11 : Delay
  cfblk12 : Delay
  cfblk3 : Subsystem  TreatAsAtomicUnit=on
  cfblk4 : Delay  DelayLengthSource=Input port
      settings: InputPortMap=u0,p1
  cfblk5 : simulink/Discrete/Tapped Delay  vinit=0.0  samptime=-1  NumDelays=1  DelayOrder=Oldest  includeCurrent=off
  cfblk6 : Delay  DelayLengthSource=Input port
      settings: InputPortMap=u0,p1
  cfblk7 : Subsystem  TreatAsAtomicUnit=on
  cfblk8 : simulink/Discrete/Transfer Fcn First Order  PoleZ=0.95  ICPrevOutput=0.0  DoSatur=off
      settings: SourceProductName=Simulink
  cyemi_{1205..1215} (11 alike) : DataTypeConversion  OutDataTypeStr=double
  emi_1190 : Subsystem  TreatAsAtomicUnit=on
  emi_1192 : If  IfExpression=0 <= u1  SampleTime=[1 0]
  emi_1193 : DataTypeConversion  OutDataTypeStr=double
  emi_1393 : Subsystem  TreatAsAtomicUnit=on
  emi_1395 : If  IfExpression=-1.586250e+00 <= u1  SampleTime=[1 0]
  emi_1396 : DataTypeConversion  OutDataTypeStr=double
  cfblk2 : Outport
  wires:
  cfblk9/1 -> cfblk2/1
  cyemi_1205/1 -> cfblk11/1
  cfblk8/1 -> cyemi_1205/1
  cyemi_1206/1 -> cfblk12/1
  cfblk6/1 -> cyemi_1206/1, emi_1396/1
  cfblk11/1 -> cyemi_1207/1, emi_1193/1
  cfblk1/1 -> cyemi_1208/1
  cyemi_1209/1 -> cfblk4/1
  cyemi_1210/1 -> cfblk4/2
  cfblk12/1 -> cyemi_1210/1
  cyemi_1211/1 -> cfblk5/1
  cyemi_1212/1 -> cfblk6/1
  cfblk5/1 -> cyemi_1212/1
  cyemi_1213/1 -> cfblk6/2
  cfblk4/1 -> cyemi_1213/1
  cfblk10/1 -> cyemi_1214/1
  cyemi_1215/1 -> cfblk8/1
  cyemi_1214/1 -> cfblk7/1(emi_1188)
  cfblk7/1(emi_1189) -> cyemi_1211/1, cyemi_1209/1
  emi_1192/1 -> cfblk7/Action
  emi_1192/2 -> emi_1190/Action
  emi_1193/1 -> emi_1192/1
  cyemi_1207/1 -> cfblk3/1(emi_1390)
  cyemi_1208/1 -> cfblk3/2(emi_1391)
  cfblk3/1(emi_1392) -> cyemi_1215/1
  emi_1395/1 -> cfblk3/Action
  emi_1395/2 -> emi_1393/Action
  emi_1396/1 -> emi_1395/1

== system sampleModel7126_pp_1_1/cfblk295 ==
  cfblk1 : Inport
  cfblk9 : Inport  Port=2
  cfblk10 : Inport  Port=3
  cfblk11 : Inport  Port=4
  Action Port : ActionPort  ActionType=then
  cfblk13 : Subsystem  TreatAsAtomicUnit=on
  cfblk14 : Subsystem  TreatAsAtomicUnit=on
  cfblk15 : Subsystem  TreatAsAtomicUnit=on
  cfblk16 : Subsystem  TreatAsAtomicUnit=on
  cfblk17 : Delay
  cfblk18 : Delay
  cfblk3 : simulink/Discrete/Difference  ICPrevInput=0.0  OutMin=[]  OutMax=[]  OutDataTypeStr=double  OutputDataTypeScalingMode=double  OutDataType=fixdt(1, 16)  OutScaling=2^-10  DoSatur=off
  cfblk4 : DiscreteFilter
  cfblk5 : Delay  DelayLengthSource=Input port
      settings: InputPortMap=u0,p1
  cfblk6 : simulink/Discrete/Transfer Fcn First Order  PoleZ=0.95  ICPrevOutput=0.0  DoSatur=off
      settings: SourceProductName=Simulink
  cfblk7 : simulink/Discrete/Transfer Fcn Real Zero  ZeroZ=0.75  ICPrevInput=0.0  DoSatur=off
      settings: SourceProductName=Simulink  SourceProductBaseCode=SL
  cfblk8 : If  SampleTime=1
  cyemi_{1220..1223,1238..1240,1255..1265} (18 alike) : DataTypeConversion  OutDataTypeStr=double
  emi_38 : Subsystem  TreatAsAtomicUnit=on
  emi_40 : If  IfExpression=Inf <= u1  SampleTime=[1 0]
  emi_41 : DataTypeConversion  OutDataTypeStr=double
  emi_706 : Subsystem  TreatAsAtomicUnit=on
  emi_708 : If  IfExpression=Inf <= u1
  emi_709 : DataTypeConversion  OutDataTypeStr=double
  cfblk2 : Outport
  cfblk12 : Outport  Port=2
  wires:
  cfblk4/1 -> cyemi_1255/1, cyemi_1264/1, emi_709/1
  cfblk5/1 -> cyemi_1258/1, cyemi_1260/1
  cfblk10/1 -> cfblk12/1
  cfblk1/1 -> cfblk2/1, cyemi_1223/1, cyemi_1240/1
  cfblk6/1 -> cyemi_1239/1, cyemi_1265/1
  cfblk8/1 -> cfblk13/Action
  cfblk8/2 -> cfblk14/Action
  cyemi_1220/1 -> cfblk13/1(cfblk1)
  cyemi_1221/1 -> cfblk13/2(cfblk15)
  cfblk17/1 -> cyemi_1221/1
  cyemi_1222/1 -> cfblk13/3(cfblk16)
  cfblk18/1 -> cyemi_1222/1, emi_41/1
  cyemi_1223/1 -> cfblk13/4(cfblk17)
  cyemi_1238/1 -> cfblk14/1(cfblk1)
  cyemi_1239/1 -> cfblk14/2(cfblk14)
  cyemi_1240/1 -> cfblk14/3(cfblk15)
  cfblk13/1(cfblk2) -> cyemi_1256/1
  cyemi_1257/1 -> cfblk17/1
  cfblk7/1 -> cyemi_1257/1
  cyemi_1258/1 -> cfblk18/1
  cyemi_1259/1 -> cfblk3/1
  cfblk11/1 -> cyemi_1259/1
  cyemi_1260/1 -> cfblk4/1
  cyemi_1261/1 -> cfblk5/1
  cfblk14/1(cfblk2) -> cyemi_1261/1
  cyemi_1262/1 -> cfblk5/2
  cfblk3/1 -> cyemi_1262/1
  cyemi_1263/1 -> cfblk6/1
  cfblk9/1 -> cyemi_1263/1
  cyemi_1264/1 -> cfblk7/1
  cyemi_1265/1 -> cfblk8/1
  cyemi_1256/1 -> cfblk16/1(emi_36)
  cfblk16/1(emi_37) -> cyemi_1238/1
  emi_40/1 -> cfblk16/Action
  emi_40/2 -> emi_38/Action
  emi_41/1 -> emi_40/1
  cyemi_1255/1 -> cfblk15/1(emi_704)
  cfblk15/1(emi_705) -> cyemi_1220/1
  emi_708/1 -> cfblk15/Action
  emi_708/2 -> emi_706/Action
  emi_709/1 -> emi_708/1

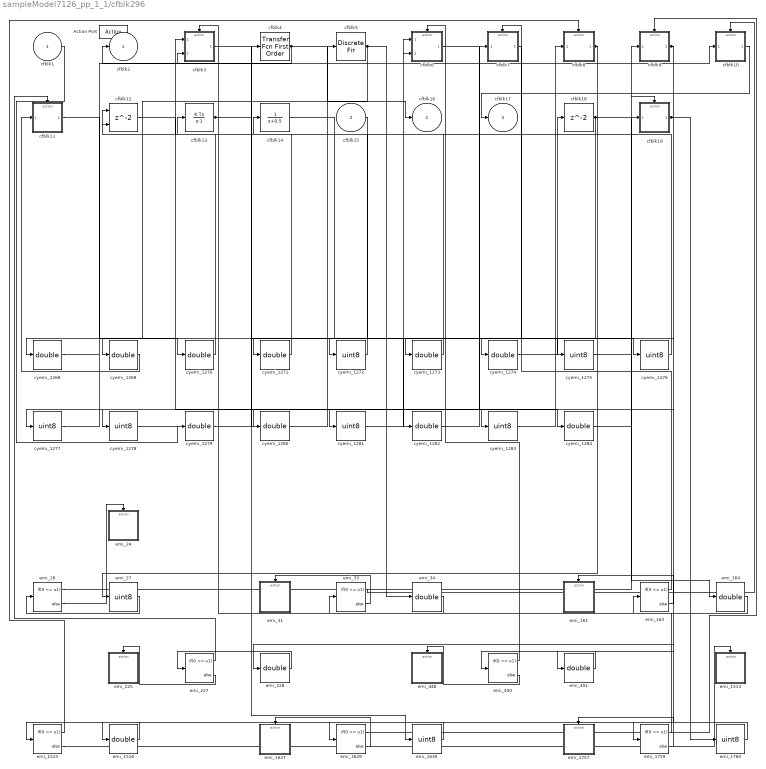
== system sampleModel7126_pp_1_1/cfblk296 ==
  cfblk1 : Inport
  cfblk15 : Inport  Port=2
  Action Port : ActionPort  ActionType=else
  cfblk10 : Subsystem  TreatAsAtomicUnit=on
  cfblk11 : Subsystem  TreatAsAtomicUnit=on
  cfblk12 : Delay  ShowEnablePort=on
      settings: InputPortMap=u0,e6
  cfblk13 : DiscreteIntegrator  SampleTime=-1  OutDataTypeStr=uint8  ICPrevOutput=DiscIntNeverNeededParam  ICPrevScaledInput=DiscIntNeverNeededParam
  cfblk14 : DiscreteTransferFcn
  cfblk18 : Delay
  cfblk19 : Subsystem  TreatAsAtomicUnit=on
  cfblk3 : Subsystem  TreatAsAtomicUnit=on
  cfblk4 : simulink/Discrete/Transfer Fcn First Order  PoleZ=0.95  ICPrevOutput=0.0  DoSatur=off
      settings: SourceProductName=Simulink
  cfblk5 : DiscreteFir
  cfblk6 : Subsystem  TreatAsAtomicUnit=on
  cfblk7 : Subsystem  TreatAsAtomicUnit=on
  cfblk8 : Subsystem  TreatAsAtomicUnit=on
  cfblk9 : Subsystem  TreatAsAtomicUnit=on
  cyemi_{1268..1271,1273..1274,1279..1280,1282,1284} (10 alike) : DataTypeConversion  OutDataTypeStr=double
  cyemi_{1272,1275..1278,1281,1283} (7 alike) : DataTypeConversion  OutDataTypeStr=uint8
  emi_1513 : Subsystem  TreatAsAtomicUnit=on
  emi_1515 : If  IfExpression=0 <= u1  SampleTime=[0 1]
  emi_{34,164,228,451,1516} (5 alike) : DataTypeConversion  OutDataTypeStr=double
  emi_161 : Subsystem  TreatAsAtomicUnit=on
  emi_1627 : Subsystem  TreatAsAtomicUnit=on
  emi_1629 : If  IfExpression=0 <= u1  SampleTime=[0 1]
  emi_163 : If  IfExpression=0 <= u1  SampleTime=[0.1 0]
  emi_1630 : DataTypeConversion  OutDataTypeStr=uint8
  emi_1757 : Subsystem  TreatAsAtomicUnit=on
  emi_1759 : If  IfExpression=0 <= u1  SampleTime=[1 0]
  emi_1760 : DataTypeConversion  OutDataTypeStr=uint8
  emi_225 : Subsystem  TreatAsAtomicUnit=on
  emi_227 : If  IfExpression=0 <= u1  SampleTime=[1 0]
  emi_24 : Subsystem  TreatAsAtomicUnit=on
  emi_26 : If  IfExpression=0 <= u1  SampleTime=[1 0]
  emi_27 : DataTypeConversion  OutDataTypeStr=uint8
  emi_31 : Subsystem  TreatAsAtomicUnit=on
  emi_33 : If  IfExpression=0 <= u1
  emi_448 : Subsystem  TreatAsAtomicUnit=on
  emi_450 : If  IfExpression=0 <= u1  SampleTime=[0.1 0]
  cfblk2 : Outport
  cfblk16 : Outport  Port=2
  cfblk17 : Outport  Port=3
  wires:
  cfblk4/1 -> cfblk2/1, cfblk16/1
  cfblk5/1 -> cyemi_1269/1, emi_34/1
  cyemi_1270/1 -> cfblk12/1
  cyemi_1271/1 -> cfblk12/2
  cfblk18/1 -> cyemi_1271/1, emi_164/1
  cyemi_1272/1 -> cfblk13/1
  cfblk15/1 -> cyemi_1272/1
  cyemi_1273/1 -> cfblk14/1
  cyemi_1274/1 -> cfblk18/1
  cfblk13/1 -> cyemi_1276/1, emi_1630/1
  cyemi_1278/1 -> cfblk4/1
  cyemi_1279/1 -> cfblk5/1
  cfblk1/1 -> cyemi_1279/1
  cfblk12/1 -> cyemi_1280/1
  cfblk14/1 -> cyemi_1282/1
  cyemi_1275/1 -> cfblk19/1(emi_22)
  cfblk19/1(emi_23) -> cyemi_1277/1, emi_1760/1
  emi_26/1 -> cfblk19/Action
  emi_26/2 -> emi_24/Action
  emi_27/1 -> emi_26/1
  cyemi_1268/1 -> cfblk10/1(emi_29)
  cfblk10/1(emi_30) -> cfblk17/1
  emi_33/1 -> cfblk10/Action
  emi_33/2 -> emi_31/Action
  emi_34/1 -> emi_33/1
  cyemi_1282/1 -> cfblk7/1(emi_159)
  cfblk7/1(emi_160) -> cyemi_1274/1
  emi_163/1 -> cfblk7/Action
  emi_163/2 -> emi_161/Action
  emi_164/1 -> emi_163/1
  cyemi_1269/1 -> cfblk11/1(emi_223)
  cfblk11/1(emi_224) -> cyemi_1270/1
  emi_227/1 -> cfblk11/Action
  emi_227/2 -> emi_225/Action
  emi_228/1 -> emi_227/1
  cyemi_1280/1 -> cfblk6/1(emi_445)
  cyemi_1281/1 -> cfblk6/2(emi_446)
  cfblk6/1(emi_447) -> cyemi_1284/1
  emi_450/1 -> cfblk6/Action
  emi_450/2 -> emi_448/Action
  emi_451/1 -> emi_450/1
  cyemi_1283/1 -> cfblk8/1(emi_1511)
  cfblk8/1(emi_1512) -> emi_27/1, cyemi_1281/1, cyemi_1278/1, cyemi_1275/1
  emi_1515/1 -> cfblk8/Action
  emi_1515/2 -> emi_1513/Action
  emi_1516/1 -> emi_1515/1
  cyemi_1284/1 -> cfblk9/1(emi_1625)
  cfblk9/1(emi_1626) -> emi_1516/1, emi_451/1, emi_228/1, cyemi_1273/1, cyemi_1268/1
  emi_1629/1 -> cfblk9/Action
  emi_1629/2 -> emi_1627/Action
  emi_1630/1 -> emi_1629/1
  cyemi_1276/1 -> cfblk3/1(emi_1754)
  cyemi_1277/1 -> cfblk3/2(emi_1755)
  cfblk3/1(emi_1756) -> cyemi_1283/1
  emi_1759/1 -> cfblk3/Action
  emi_1759/2 -> emi_1757/Action
  emi_1760/1 -> emi_1759/1

== system sampleModel7126_pp_1_1/cfblk297 ==
  cfblk1 : Inport
  cfblk8 : Inport  Port=2
  cfblk9 : Inport  Port=3
  Action Port : ActionPort  ActionType=then
  cfblk11 : Delay
  cfblk3 : DiscreteFilter
  cfblk4 : simulink/Discrete/Tapped Delay  vinit=0.0  samptime=-1  NumDelays=1  DelayOrder=Oldest  includeCurrent=off
  cfblk5 : simulink/Continuous/PID Controller  Controller=PID  TimeDomain=Discrete-time  SampleTime=-1  IntegratorMethod=Forward Euler  FilterMethod=Forward Euler  Form=Parallel  UseFilter=on  ControllerParametersSource=internal  P=1  I=1  D=0  N=100  InitialConditionSource=internal  InitialConditionForIntegrator=0  InitialConditionForFilter=0  ExternalReset=none  LimitOutput=off  UpperSaturationLimit=inf  LowerSaturationLimit=-inf  LinearizeAsGain=off  AntiWindupMode=none  Kb=1  TrackingMode=off  Kt=1  PParamMin=[]  PParamMax=[]  IParamMin=[]  IParamMax=[]  DParamMin=[]  DParamMax=[]  NParamMin=[]  NParamMax=[]  KbParamMin=[]  KbParamMax=[]  KtParamMin=[]  KtParamMax=[]  POutMin=[]  POutMax=[]  IOutMin=[]  IOutMax=[]  DOutMin=[]  DOutMax=[]  NOutMin=[]  NOutMax=[]  KbOutMin=[]  KbOutMax=[]  KtOutMin=[]  KtOutMax=[]  IntegratorOutMin=[]  IntegratorOutMax=[]  FilterOutMin=[]  FilterOutMax=[]  SumOutMin=[]  SumOutMax=[]  SumI1OutMin=[]  SumI1OutMax=[]  SumI2OutMin=[]  SumI2OutMax=[]  SumI3OutMin=[]  SumI3OutMax=[]  SumDOutMin=[]  SumDOutMax=[]  SaturationOutMin=[]  SaturationOutMax=[]  IntegratorContinuousStateAttributes=''  IntegratorStateMustResolveToSignalObject=off  IntegratorRTWStateStorageClass=Auto  FilterContinuousStateAttributes=''  FilterStateMustResolveToSignalObject=off  FilterRTWStateStorageClass=Auto  DifferentiatorICPrevScaledInput=0  DifferentiatorOutMin=[]  DifferentiatorOutMax=[]  FilterDiffOutCoefMin=[]  FilterDiffOutCoefMax=[]  SumDenOutMin=[]  SumDenOutMax=[]  SumNumOutMin=[]  SumNumOutMax=[]  ReciprocalOutMin=[]  ReciprocalOutMax=[]  DivideOutMin=[]  DivideOutMax=[]  TunerSelectOption=Transfer Function Based (PID Tuner App)
  cfblk6 : simulink/Discrete/Difference  ICPrevInput=0.0  OutMin=[]  OutMax=[]  OutDataTypeStr=double  OutputDataTypeScalingMode=double  OutDataType=fixdt(1, 16)  OutScaling=2^-10  DoSatur=off
  cfblk7 : Subsystem  TreatAsAtomicUnit=on
  cyemi_{1288..1294} (7 alike) : DataTypeConversion  OutDataTypeStr=double
  emi_2032 : Subsystem  TreatAsAtomicUnit=on
  emi_2034 : If  IfExpression=Inf <= u1  SampleTime=[1 0]
  emi_2035 : DataTypeConversion  OutDataTypeStr=double
  cfblk2 : Outport
  cfblk10 : Outport  Port=2
  wires:
  cfblk1/1 -> cfblk10/1
  cfblk6/1 -> cfblk2/1
  cyemi_1288/1 -> cfblk11/1
  cyemi_1289/1 -> cfblk3/1
  cfblk11/1 -> cyemi_1289/1
  cyemi_1290/1 -> cfblk4/1
  cfblk9/1 -> cyemi_1290/1
  cyemi_1291/1 -> cfblk5/1
  cfblk8/1 -> cyemi_1291/1
  cyemi_1292/1 -> cfblk6/1
  cfblk4/1 -> cyemi_1292/1, emi_2035/1
  cfblk5/1 -> cyemi_1293/1
  cfblk3/1 -> cyemi_1294/1
  cyemi_1293/1 -> cfblk7/1(emi_2029)
  cyemi_1294/1 -> cfblk7/2(emi_2030)
  cfblk7/1(emi_2031) -> cyemi_1288/1
  emi_2034/1 -> cfblk7/Action
  emi_2034/2 -> emi_2032/Action
  emi_2035/1 -> emi_2034/1

== system sampleModel7126_pp_1_1/cfblk298 ==
  cfblk1 : Inport
  cfblk9 : Inport  Port=2
  cfblk10 : Inport  Port=3
  cfblk11 : Inport  Port=4
  Action Port : ActionPort  ActionType=else
  cfblk15 : Subsystem  TreatAsAtomicUnit=on
  cfblk16 : Subsystem  TreatAsAtomicUnit=on
  cfblk17 : Delay
  cfblk18 : Delay
  cfblk19 : Delay
  cfblk3 : Subsystem  TreatAsAtomicUnit=on
  cfblk4 : Subsystem  TreatAsAtomicUnit=on
  cfblk5 : DiscreteZeroPole  Poles=[0 0.5]  Gain=1  SampleTime=-1
  cfblk6 : DiscreteZeroPole  Poles=[0 0.5]  Gain=1  SampleTime=-1
  cfblk7 : DiscreteFilter
  cfblk8 : If  SampleTime=1
  cyemi_{1299..1300,1314,1331..1339} (12 alike) : DataTypeConversion  OutDataTypeStr=double
  emi_1293 : Subsystem  TreatAsAtomicUnit=on
  emi_1295 : If  IfExpression=0 <= u1  SampleTime=[1 0]
  emi_1296 : DataTypeConversion  OutDataTypeStr=double
  emi_1705 : Subsystem  TreatAsAtomicUnit=on
  emi_1707 : If  IfExpression=0 <= u1  SampleTime=[1 0]
  emi_1708 : DataTypeConversion  OutDataTypeStr=double
  cfblk2 : Outport
  cfblk12 : Outport  Port=2
  cfblk13 : Outport  Port=3
  cfblk14 : Outport  Port=4
  wires:
  cfblk10/1 -> cfblk14/1
  cfblk15/1(cfblk2) -> cfblk12/1
  cfblk9/1 -> cfblk13/1
  cfblk8/1 -> cfblk15/Action
  cfblk8/2 -> cfblk16/Action
  cyemi_1299/1 -> cfblk15/1(cfblk1)
  cfblk11/1 -> cyemi_1299/1, cyemi_1300/1
  cyemi_1300/1 -> cfblk15/2(cfblk14)
  cyemi_1314/1 -> cfblk16/1(cfblk1)
  cfblk7/1 -> cyemi_1314/1
  cyemi_1331/1 -> cfblk17/1
  cfblk6/1 -> cyemi_1331/1, emi_1708/1
  cyemi_1332/1 -> cfblk18/1
  cfblk16/1(cfblk2) -> cyemi_1332/1
  cyemi_1333/1 -> cfblk19/1
  cfblk15/2(cfblk15) -> cyemi_1333/1
  cfblk17/1 -> cyemi_1334/1
  cfblk1/1 -> cyemi_1335/1
  cyemi_1336/1 -> cfblk5/1
  cfblk18/1 -> cyemi_1336/1, emi_1296/1
  cyemi_1337/1 -> cfblk6/1
  cyemi_1338/1 -> cfblk7/1
  cfblk5/1 -> cyemi_1338/1
  cyemi_1339/1 -> cfblk8/1
  cfblk19/1 -> cyemi_1339/1
  cyemi_1335/1 -> cfblk4/1(emi_1291)
  cfblk4/1(emi_1292) -> cfblk2/1
  emi_1295/1 -> cfblk4/Action
  emi_1295/2 -> emi_1293/Action
  emi_1296/1 -> emi_1295/1
  cyemi_1334/1 -> cfblk3/1(emi_1703)
  cfblk3/1(emi_1704) -> cyemi_1337/1
  emi_1707/1 -> cfblk3/Action
  emi_1707/2 -> emi_1705/Action
  emi_1708/1 -> emi_1707/1

== system sampleModel7126_pp_1_1/cfblk319 ==
  emi_1660 : Inport
  Action Port : ActionPort  ActionType=then
  cfblk319 : Delay  SampleTime=1
  emi_1661 : Outport
  wires:
  emi_1660/1 -> cfblk319/1
  cfblk319/1 -> emi_1661/1

== system sampleModel7126_pp_1_1/cfblk325 ==
  emi_1834 : Inport
  Action Port : ActionPort  ActionType=then
  cfblk325 : Delay  SampleTime=1
  emi_1835 : Outport
  wires:
  emi_1834/1 -> cfblk325/1
  cfblk325/1 -> emi_1835/1

== system sampleModel7126_pp_1_1/cfblk33 ==
  emi_1419 : Inport
  Action Port : ActionPort  ActionType=then
  cfblk33 : Delay  SampleTime=1
  emi_1420 : Outport
  wires:
  emi_1419/1 -> cfblk33/1
  cfblk33/1 -> emi_1420/1

== system sampleModel7126_pp_1_1/cfblk332 ==
  emi_1806 : Inport
  Action Port : ActionPort  ActionType=then
  cfblk332 : Delay  SampleTime=1
  emi_1807 : Outport
  wires:
  emi_1806/1 -> cfblk332/1
  cfblk332/1 -> emi_1807/1

== system sampleModel7126_pp_1_1/cfblk334 ==
  emi_825 : Inport
  Action Port : ActionPort  ActionType=then
  cfblk334 : Delay  SampleTime=1
  emi_826 : Outport
  wires:
  emi_825/1 -> cfblk334/1
  cfblk334/1 -> emi_826/1

== system sampleModel7126_pp_1_1/cfblk337 ==
  emi_2102 : Inport
  Action Port : ActionPort  ActionType=then
  cfblk337 : Delay  SampleTime=1
  emi_2103 : Outport
  wires:
  emi_2102/1 -> cfblk337/1
  cfblk337/1 -> emi_2103/1

== system sampleModel7126_pp_1_1/cfblk338 ==
  emi_1827 : Inport
  Action Port : ActionPort  ActionType=then
  cfblk338 : Delay  SampleTime=1
  emi_1828 : Outport
  wires:
  emi_1827/1 -> cfblk338/1
  cfblk338/1 -> emi_1828/1

== system sampleModel7126_pp_1_1/cfblk340 ==
  emi_1081 : Inport
  Action Port : ActionPort  ActionType=then
  cfblk340 : Delay  SampleTime=1
  emi_1082 : Outport
  wires:
  emi_1081/1 -> cfblk340/1
  cfblk340/1 -> emi_1082/1

== system sampleModel7126_pp_1_1/cfblk342 ==
  emi_796 : Inport
  Action Port : ActionPort  ActionType=then
  cfblk342 : Delay  SampleTime=1
  emi_797 : Outport
  wires:
  emi_796/1 -> cfblk342/1
  cfblk342/1 -> emi_797/1

== system sampleModel7126_pp_1_1/cfblk347 ==
  emi_187 : Inport
  Action Port : ActionPort  ActionType=then
  cfblk347 : Delay  SampleTime=1
  emi_188 : Outport
  wires:
  emi_187/1 -> cfblk347/1
  cfblk347/1 -> emi_188/1

== system sampleModel7126_pp_1_1/cfblk37 ==
  emi_1532 : Inport
  emi_1533 : Inport  Port=2
  Action Port : ActionPort  ActionType=then
  cfblk37 : Delay  ShowEnablePort=on  SampleTime=1
      settings: InputPortMap=u0,e6
  emi_1534 : Outport
  wires:
  emi_1532/1 -> cfblk37/1
  emi_1533/1 -> cfblk37/2
  cfblk37/1 -> emi_1534/1

== system sampleModel7126_pp_1_1/cfblk39 ==
  emi_789 : Inport
  Action Port : ActionPort  ActionType=then
  cfblk39 : DiscreteTransferFcn  SampleTime=1
  emi_790 : Outport
  wires:
  emi_789/1 -> cfblk39/1
  cfblk39/1 -> emi_790/1
